simulink model "test_mdl"  (R2023a)
settings: Solver=VariableStepAuto  StartTime=0.0  StopTime=10.0  RelTol=1e-3
settings Model: Creator=smqwzy  LastModifiedBy=smqwzy

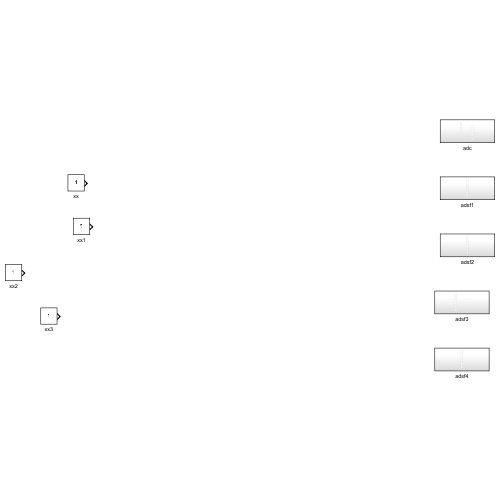
[thumbnail: Simulink's stored preview of the top-level diagram]
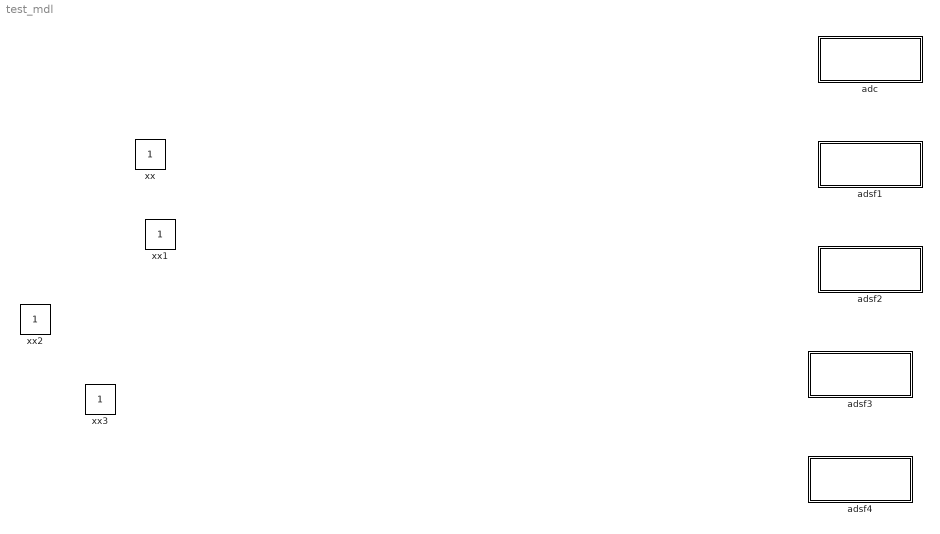
== system test_mdl ==
  adc : Subsystem
  adsf1 : Subsystem
  adsf2 : Subsystem
  adsf3 : Subsystem
  adsf4 : Subsystem
  xx{,1..3} (4 alike) : Constant

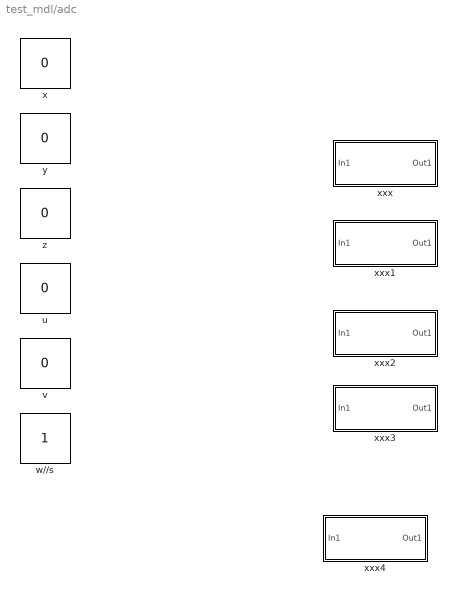
== system test_mdl/adc ==
  u : Constant  Value=0
  v : Constant  Value=0
  w//s : Constant
  x : Constant  Value=0
  xxx : Subsystem
  xxx1 : Subsystem
  xxx2 : Subsystem
  xxx3 : Subsystem
  xxx4 : Subsystem
  y : Constant  Value=0
  z : Constant  Value=0

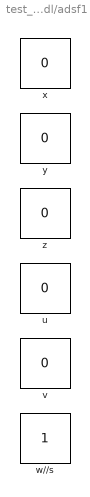
== system test_mdl/adsf1 ==
  u : Constant  Value=0
  v : Constant  Value=0
  w//s : Constant
  x : Constant  Value=0
  y : Constant  Value=0
  z : Constant  Value=0

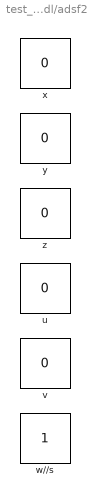
== system test_mdl/adsf2 ==
  u : Constant  Value=0
  v : Constant  Value=0
  w//s : Constant
  x : Constant  Value=0
  y : Constant  Value=0
  z : Constant  Value=0

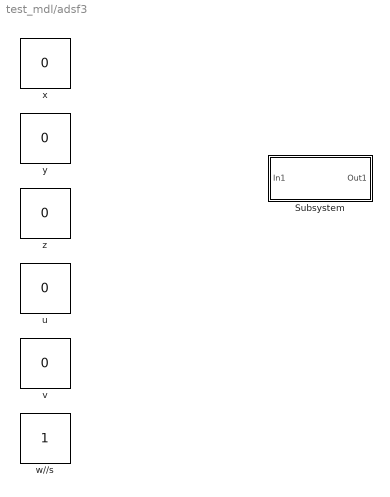
== system test_mdl/adsf3 ==
  Subsystem : Subsystem
  u : Constant  Value=0
  v : Constant  Value=0
  w//s : Constant
  x : Constant  Value=0
  y : Constant  Value=0
  z : Constant  Value=0

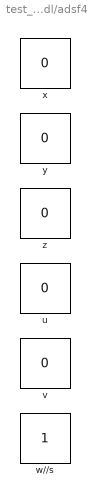
== system test_mdl/adsf4 ==
  u : Constant  Value=0
  v : Constant  Value=0
  w//s : Constant
  x : Constant  Value=0
  y : Constant  Value=0
  z : Constant  Value=0

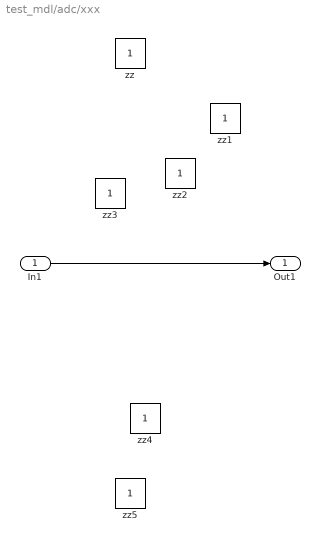
== system test_mdl/adc/xxx ==
  In1 : Inport
  zz{,1..5} (6 alike) : Constant
  Out1 : Outport
  wires:
  In1/1 -> Out1/1

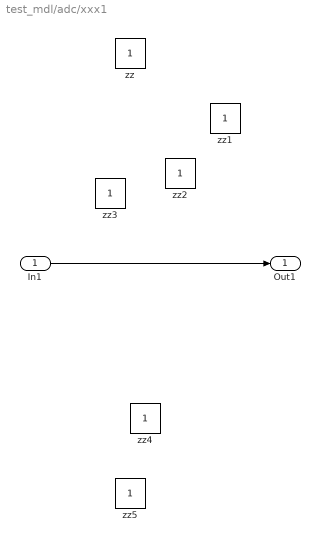
== system test_mdl/adc/xxx1 ==
  In1 : Inport
  zz{,1..5} (6 alike) : Constant
  Out1 : Outport
  wires:
  In1/1 -> Out1/1

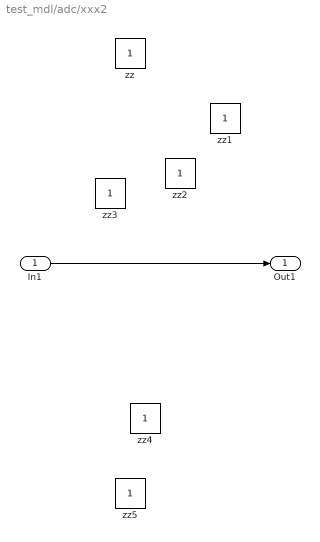
== system test_mdl/adc/xxx2 ==
  In1 : Inport
  zz{,1..5} (6 alike) : Constant
  Out1 : Outport
  wires:
  In1/1 -> Out1/1

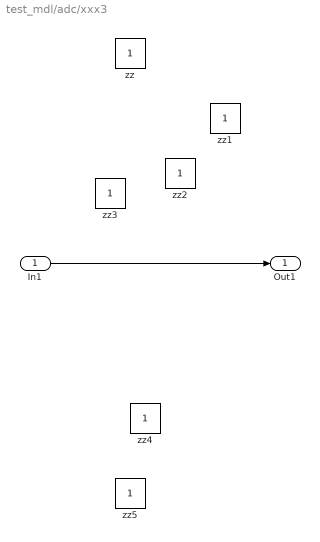
== system test_mdl/adc/xxx3 ==
  In1 : Inport
  zz{,1..5} (6 alike) : Constant
  Out1 : Outport
  wires:
  In1/1 -> Out1/1

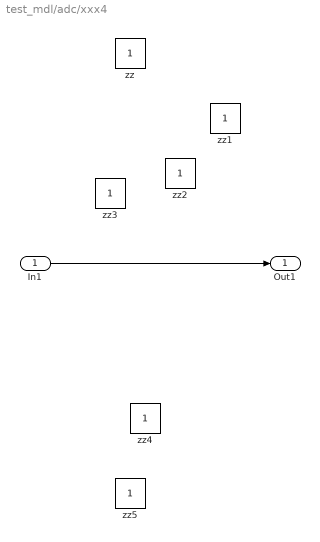
== system test_mdl/adc/xxx4 ==
  In1 : Inport
  zz{,1..5} (6 alike) : Constant
  Out1 : Outport
  wires:
  In1/1 -> Out1/1

== system test_mdl/adsf3/Subsystem ==
  In1 : Inport
  xxx : Subsystem
  Out1 : Outport
  wires:
  In1/1 -> Out1/1

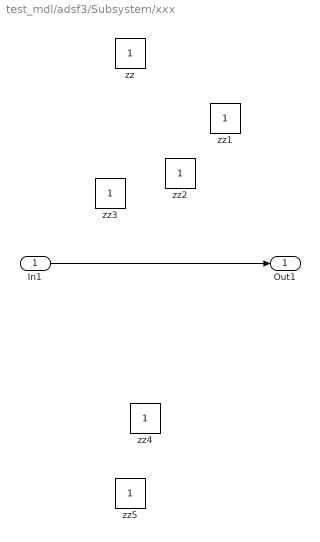
== system test_mdl/adsf3/Subsystem/xxx ==
  In1 : Inport
  zz{,1..5} (6 alike) : Constant
  Out1 : Outport
  wires:
  In1/1 -> Out1/1
